simulink model "Problem_Iz"  (R2020b)
settings: Solver=VariableStepAuto  StartTime=0.0  StopTime=Ts  RelTol=1e-3
PreLoadFcn:
  | setUpPurePursuitCurveHighVel
model workspace (MAT data in the model file):
  firstWarning = 0
  originalScenarioChecksum = 'F73A6DA3C723D3CA73A6F931B7A52A9C'
values from neighbouring files (symbols this model uses):
  Cf = 34282    [matlab.mat]    (also in matlab2.mat)
  Cr = 34282    [matlab.mat]    (also in matlab2.mat)
  g = 9.81    [matlab.mat]    (also in matlab2.mat)
  i = 5.45    [matlab.mat]    (also in matlab2.mat)
  Iz = 162    [matlab.mat]    (also in matlab2.mat)
  L = 1.524    [matlab.mat]    (also in matlab2.mat)
  ld = 2    [matlab.mat]    (also in matlab2.mat)
  lf = 0.686    [matlab.mat]    (also in matlab2.mat)
  lr = 0.838    [matlab.mat]    (also in matlab2.mat)
  m = 300    [matlab.mat]    (also in matlab2.mat)
  Rw = 0.265    [matlab.mat]    (also in matlab2.mat)
  s = [73 1]    [matlab.mat]    (also in matlab2.mat)
  tr = 0.549    [matlab.mat]    (also in matlab2.mat)
  X_o = 0    [matlab.mat]    (also in matlab2.mat)
  xRef = [0 1.324067355 2.607903593 3.8125 4.901255524 5.841088879 6.603443704 7.165156233 7.509159117 7.625 7.509159117 7.165156233 ... (73 elements, 73x1)]    [matlab.mat]    (also in matlab2.mat)
  Y_o = 0    [matlab.mat]    (also in matlab2.mat)
  yRef = [0 0.115840883 0.459843767 1.021556296 1.783911121 2.723744476 3.8125 5.017096407 6.300932645 7.625 8.949067355 10.23290359 ... (73 elements, 73x1)]    [matlab.mat]    (also in matlab2.mat)
undefined symbols (not defined in the file or in its folder): psi_o, sigma1
libraries: autolibutils x4, autolibshared x3, simulink x3, pid_lib x2, vehdynlibviscommon x1, robotalgslib x1
(part 3 of 3)

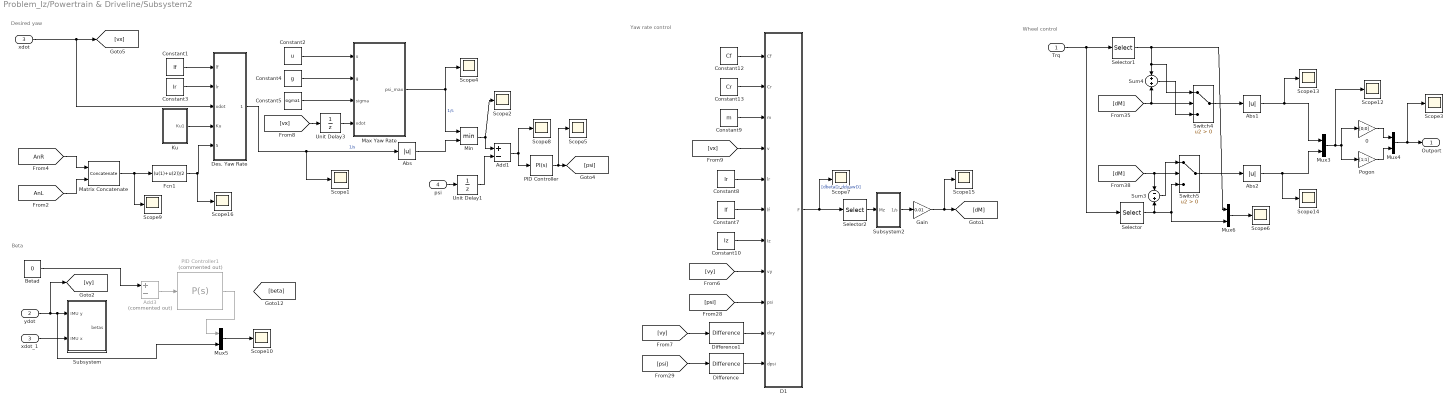
== system Problem_Iz/Powertrain & Driveline/Subsystem2 ==
  note: Desired yaw
  note: Beta
  note: Yaw rate control
  note: Wheel control
  Trq : Inport
  ydot : Inport  Port=2
  xdot : Inport  Port=3
  psi : Inport  Port=4
  0 : Gain  Gain=[0;0]
  Abs : Abs
  Abs1 : Abs
  Abs2 : Abs
  Add1 : Sum  Inputs=+-
  Add3 : Sum  Commented=on  Inputs=+-
  Betad : Constant  Value=0
  Constant1 : Constant  Value=lf
  Constant10 : Constant  Value=Iz
  Constant12 : Constant  Value=Cf
  Constant13 : Constant  Value=Cr
  Constant2 : Constant  Value=u
  Constant3 : Constant  Value=lr
  Constant4 : Constant  Value=g
  Constant5 : Constant  Value=sigma1
  Constant7 : Constant  Value=lf
  Constant8 : Constant  Value=lr
  Constant9 : Constant  Value=m
  D1 : MATLAB Function  TreatAsAtomicUnit=on
  Des. Yaw Rate : MATLAB Function  TreatAsAtomicUnit=on
  Difference : simulink/Discrete/Difference  ICPrevInput=0.0  OutMin=[]  OutMax=[]  OutDataType=fixdt(1, 16)  OutScaling=2^-10  DoSatur=off
  Difference1 : simulink/Discrete/Difference  ICPrevInput=0.0  OutMin=[]  OutMax=[]  OutDataType=fixdt(1, 16)  OutScaling=2^-10  DoSatur=off
  Fcn1 : Fcn  Expr=(u(1)+u(2))/2
  Gain : Gain  Gain=0.01
  Ku : Subsystem
  Matrix Concatenate : Concatenate
  Max Yaw Rate : MATLAB Function  TreatAsAtomicUnit=on
  Min : MinMax  Inputs=2
  Mux{3..6} (4 alike) : Mux  Inputs=2
  PID Controller : pid_lib/PID Controller  Controller=PI  Form=Parallel  TimeDomain=Continuous-time  UseExternalTs=off  SampleTime=-1  IntegratorMethod=Forward Euler  FilterMethod=Forward Euler  ControllerParametersSource=internal  P=4  I=12.5  D=0  UseFilter=on  N=100  TunerSelectOption=Transfer Function Based (PID Tuner App)  InitialConditionSource=internal  InitialConditionForIntegrator=0  InitialConditionForFilter=0  DifferentiatorICPrevScaledInput=0  ExternalReset=none  TrackingMode=off  Kt=1  LimitOutput=off  SatLimitsSource=internal  UpperSaturationLimit=inf  LowerSaturationLimit=-inf  LinearizeAsGain=on  AntiWindupMode=none  Kb=1  POutMin=[]  POutMax=[]  IOutMin=[]  IOutMax=[]  DOutMin=[]  DOutMax=[]  NOutMin=[]  NOutMax=[]  SumOutMin=[]  SumOutMax=[]  SaturationOutMin=[]  SaturationOutMax=[]  PParamMin=[]  PParamMax=[]  IParamMin=[]  IParamMax=[]  DParamMin=[]  DParamMax=[]  NParamMin=[]  NParamMax=[]  KbParamMin=[]  KbParamMax=[]  KtParamMin=[]  KtParamMax=[]  KbOutMin=[]  KbOutMax=[]  KtOutMin=[]  KtOutMax=[]  IntegratorOutMin=[]  IntegratorOutMax=[]  FilterOutMin=[]  FilterOutMax=[]  SumI1OutMin=[]  SumI1OutMax=[]  SumI2OutMin=[]  SumI2OutMax=[]  SumI3OutMin=[]  SumI3OutMax=[]  SumI4OutMin=[]  SumI4OutMax=[]  SumDOutMin=[]  SumDOutMax=[]  DifferentiatorOutMin=[]  DifferentiatorOutMax=[]  FilterDiffOutCoefMin=[]  FilterDiffOutCoefMax=[]  ReciprocalOutMin=[]  ReciprocalOutMax=[]  SumDenOutMin=[]  SumDenOutMax=[]  SumNumOutMin=[]  SumNumOutMax=[]  DivideOutMin=[]  DivideOutMax=[]  UdiffTsProdOutMin=[]  UdiffTsProdOutMax=[]  NTsProdOutMin=[]  NTsProdOutMax=[]  UintegralTsProdOutMin=[]  UintegralTsProdOutMax=[]  UngainTsProdOutMin=[]  UngainTsProdOutMax=[]  IntegratorContinuousStateAttributes=''  IntegratorStateMustResolveToSignalObject=off  IntegratorRTWStateStorageClass=Auto  FilterContinuousStateAttributes=''  FilterStateMustResolveToSignalObject=off  FilterRTWStateStorageClass=Auto  ParallelPVariant=InternalParameters  IdealPVariant=Disabled  IVariant=InternalParameters  DVariant=Disabled  IntegratorVariant=Continuous  SatVariant=Disabled  AWVariant=Passthrough  PCopyVariant=Disabled  TRVariant=Disabled  FdbkBlocksVariant=Forward  IdealPFdbkVariant=Disabled  SatFdbkVariant=Disabled  DerivativeFilterVariant=Disabled  NVariant=Disabled  NCopyVariant=Disabled_SignalSpec  FilterICVariant=Disabled  IntegratorICVariant=InternalICs  ExternalResetVariant=Disabled  TRSumVariant=Passthrough  SumFdbkVariant=Disabled  SumVariant=Sum_PI  TsampFilterVariant=InternalTs  TsampNgainVariant=Passthrough  TsampIntegralVariant=Passthrough  ExternalSaturationOutDataTypeStr=Inherit: Same as second input
  PID Controller1 : pid_lib/PID Controller  Commented=on  Controller=P  Form=Parallel  TimeDomain=Continuous-time  UseExternalTs=off  SampleTime=-1  IntegratorMethod=Forward Euler  FilterMethod=Forward Euler  ControllerParametersSource=internal  P=1  I=0.001  D=0  UseFilter=on  N=100  TunerSelectOption=Transfer Function Based (PID Tuner App)  InitialConditionSource=internal  InitialConditionForIntegrator=0  InitialConditionForFilter=0  DifferentiatorICPrevScaledInput=0  ExternalReset=none  TrackingMode=off  Kt=1  LimitOutput=off  SatLimitsSource=internal  UpperSaturationLimit=inf  LowerSaturationLimit=-inf  LinearizeAsGain=on  AntiWindupMode=none  Kb=1  POutMin=[]  POutMax=[]  IOutMin=[]  IOutMax=[]  DOutMin=[]  DOutMax=[]  NOutMin=[]  NOutMax=[]  SumOutMin=[]  SumOutMax=[]  SaturationOutMin=[]  SaturationOutMax=[]  PParamMin=[]  PParamMax=[]  IParamMin=[]  IParamMax=[]  DParamMin=[]  DParamMax=[]  NParamMin=[]  NParamMax=[]  KbParamMin=[]  KbParamMax=[]  KtParamMin=[]  KtParamMax=[]  KbOutMin=[]  KbOutMax=[]  KtOutMin=[]  KtOutMax=[]  IntegratorOutMin=[]  IntegratorOutMax=[]  FilterOutMin=[]  FilterOutMax=[]  SumI1OutMin=[]  SumI1OutMax=[]  SumI2OutMin=[]  SumI2OutMax=[]  SumI3OutMin=[]  SumI3OutMax=[]  SumI4OutMin=[]  SumI4OutMax=[]  SumDOutMin=[]  SumDOutMax=[]  DifferentiatorOutMin=[]  DifferentiatorOutMax=[]  FilterDiffOutCoefMin=[]  FilterDiffOutCoefMax=[]  ReciprocalOutMin=[]  ReciprocalOutMax=[]  SumDenOutMin=[]  SumDenOutMax=[]  SumNumOutMin=[]  SumNumOutMax=[]  DivideOutMin=[]  DivideOutMax=[]  UdiffTsProdOutMin=[]  UdiffTsProdOutMax=[]  NTsProdOutMin=[]  NTsProdOutMax=[]  UintegralTsProdOutMin=[]  UintegralTsProdOutMax=[]  UngainTsProdOutMin=[]  UngainTsProdOutMax=[]  IntegratorContinuousStateAttributes=''  IntegratorStateMustResolveToSignalObject=off  IntegratorRTWStateStorageClass=Auto  FilterContinuousStateAttributes=''  FilterStateMustResolveToSignalObject=off  FilterRTWStateStorageClass=Auto  ParallelPVariant=InternalParameters  IdealPVariant=Disabled  IVariant=Disabled  DVariant=Disabled  IntegratorVariant=Disabled  SatVariant=Disabled  AWVariant=Disabled  PCopyVariant=Disabled  TRVariant=Disabled  FdbkBlocksVariant=Forward  IdealPFdbkVariant=Disabled  SatFdbkVariant=Disabled  DerivativeFilterVariant=Disabled  NVariant=Disabled  NCopyVariant=Disabled_SignalSpec  FilterICVariant=Disabled  IntegratorICVariant=Disabled  ExternalResetVariant=Disabled  TRSumVariant=Passthrough  SumFdbkVariant=Disabled  SumVariant=Passthrough_P  TsampFilterVariant=InternalTs  TsampNgainVariant=Passthrough  TsampIntegralVariant=Disabled_SignalSpec  ExternalSaturationOutDataTypeStr=Inherit: Same as second input
  Pogon : Gain  Gain=[1;1]
  Scope{1..10,12..16} (15 alike) : Scope
  Selector : Selector  InputPortWidth=4  IndexOptions=Index vector (dialog)  Indices=[4 ]  OutputSizes=1
  Selector1 : Selector  InputPortWidth=4  IndexOptions=Index vector (dialog)  Indices=[3]  OutputSizes=1
  Selector2 : Selector  InputPortWidth=2  IndexOptions=Index vector (dialog)  Indices=[1]  OutputSizes=1
  Subsystem : Subsystem
  Subsystem2 : Subsystem
  Sum3 : Sum  Inputs=-+
  Sum4 : Sum
  Switch4 : Switch  Criteria=u2 > Threshold
  Switch5 : Switch  Criteria=u2 > Threshold
  Unit Delay1 : UnitDelay  SampleTime=0.7  HasFrameUpgradeWarning=on
  Unit Delay3 : UnitDelay  SampleTime=0.7  HasFrameUpgradeWarning=on
  xdot_1 : InportShadow  Port=3
  Outport : Outport
  wires:
  [psi] -> D1/9(psi)
  [AnR] -> Matrix Concatenate/1
  Constant12/1 -> D1/1(Cf)
  Trq/1 -> Selector/1, Selector1/1
  xdot/1 -> [vx], Des. Yaw Rate/3(xdot)
  [AnL] -> Matrix Concatenate/2
  Constant3/1 -> Des. Yaw Rate/2(lr)
  psi/1 -> Unit Delay1/1
  Constant4/1 -> Max Yaw Rate/2(g)
  [vy] -> Difference1/1
  Des. Yaw Rate/1(psi_des) -> Abs/1, Scope1/1  "1/s"
  [vx] -> D1/4(v)
  Constant2/1 -> Max Yaw Rate/1(u)
  Mux3/1 -> Scope12/1, 0/1, Pogon/1
  Matrix Concatenate/1 -> Scope9/1, Fcn1/1
  D1/1(F) -> Selector2/1, Scope7/1  "[dbetaD; ddyawD]"
  Constant5/1 -> Max Yaw Rate/3(sigma)
  [psi] -> Difference/1
  Switch5/1 -> Abs2/1
  Min/1 -> Add1/1, Scope2/1
  [dM] -> Switch5/2, Sum3/1
  Sum3/1 -> Switch5/1
  Mux4/1 -> Outport/1, Scope3/1
  Constant13/1 -> D1/2(Cr)
  Constant8/1 -> D1/5(lr)
  Constant9/1 -> D1/3(m)
  Constant7/1 -> D1/6(lf)
  0/1 -> Mux4/1
  Constant1/1 -> Des. Yaw Rate/1(lf)
  Fcn1/1 -> Scope16/1, Des. Yaw Rate/5(WhiAngF)
  Betad/1 -> Add3/1
  PID Controller/1 -> Scope5/1, [psi]
  [dM] -> Sum4/2, Switch4/2
  Max Yaw Rate/1(psi_max) -> Min/1, Scope4/1  "1/s"
  [vy] -> D1/8(vy)
  Selector/1 -> Mux6/2, Switch5/3, Sum3/2
  PID Controller1/1 -> Mux5/1
  Sum4/1 -> Switch4/3
  Ku/1(Ku1) -> Des. Yaw Rate/4(Ku)
  ydot/1 -> [vy], Mux5/2, Subsystem/1(IMU y)
  Constant10/1 -> D1/7(Iz)
  Add3/1 -> PID Controller1/1
  [vx] -> Unit Delay3/1
  xdot_1/1 -> Subsystem/2(IMU x)
  Pogon/1 -> Mux4/2
  Selector1/1 -> Mux6/1, Switch4/1, Sum4/1
  Switch4/1 -> Abs1/1
  Mux5/1 -> Scope10/1
  Mux6/1 -> Scope6/1
  Unit Delay3/1 -> Max Yaw Rate/4(xdot)
  Add1/1 -> Scope8/1, PID Controller/1
  Abs/1 -> Min/2
  Difference1/1 -> D1/10(dvy)
  Difference/1 -> D1/11(dpsi)
  Selector2/1 -> Subsystem2/1(Mz)
  Unit Delay1/1 -> Add1/2
  Subsystem2/1(1/s) -> Gain/1
  Abs1/1 -> Mux3/1, Scope13/1
  Abs2/1 -> Scope14/1, Mux3/2
  Gain/1 -> Scope15/1, [dM]

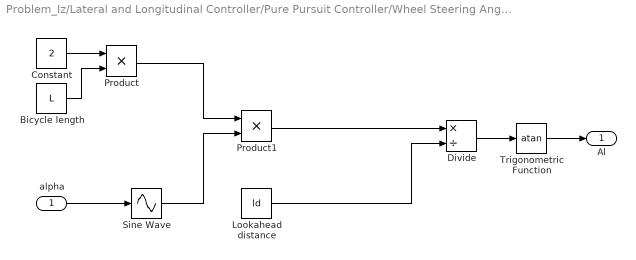
== system Problem_Iz/Lateral and Longitudinal Controller/Pure Pursuit Controller/Wheel Steering Angle Formulation ==
  alpha : Inport
  Bicycle length : Constant  Value=L
  Constant : Constant  Value=2
  Divide : Product  Inputs=*/
  Lookahead distance : Constant  Value=ld
  Product : Product
  Product1 : Product
  Sine Wave : Sin  TimeSource=Use external signal  SampleTime=0
  Trigonometric Function : Trigonometry  Operator=atan
  Al : Outport
  wires:
  Sine Wave/1 -> Product1/2
  Bicycle length/1 -> Product/2
  Constant/1 -> Product/1
  Product1/1 -> Divide/1
  Product/1 -> Product1/1
  Divide/1 -> Trigonometric Function/1
  Trigonometric Function/1 -> Al/1
  alpha/1 -> Sine Wave/1
  Lookahead distance/1 -> Divide/2

== system Problem_Iz/Powertrain & Driveline/Driveline/RWD ==
  TPowertrain : Inport
  RWD : Gain  Gain=[0;0;1;1]
  TAxles : Outport  VectorParamsAs1DForOutWhenUnconnected=off
  wires:
  TPowertrain/1 -> RWD/1
  RWD/1 -> TAxles/1

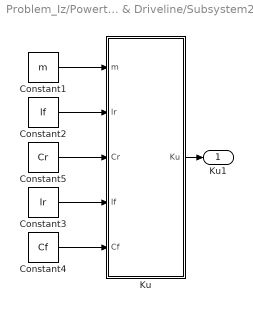
== system Problem_Iz/Powertrain & Driveline/Subsystem2/Ku ==
  Constant1 : Constant  Value=m
  Constant2 : Constant  Value=lf
  Constant3 : Constant  Value=lr
  Constant4 : Constant  Value=Cf
  Constant5 : Constant  Value=Cr
  Ku : MATLAB Function  TreatAsAtomicUnit=on
  Ku1 : Outport
  wires:
  Ku/1(Ku) -> Ku1/1
  Constant5/1 -> Ku/3(Cr)
  Constant2/1 -> Ku/2(lr)
  Constant3/1 -> Ku/4(lf)
  Constant1/1 -> Ku/1(m)
  Constant4/1 -> Ku/5(Cf)

== system Problem_Iz/Powertrain & Driveline/Subsystem2/Subsystem ==
  IMU y : Inport
  IMU x : Inport  Port=2
  Betas : Product  Inputs=*/
  Scope1 : Scope
  Tan : Trigonometry  Operator=atan
  betas : Outport
  wires:
  IMU y/1 -> Betas/1
  IMU x/1 -> Betas/2
  Betas/1 -> Tan/1
  Tan/1 -> Scope1/1, betas/1

== system Problem_Iz/Powertrain & Driveline/Subsystem2/Subsystem2 ==
  Mz : Inport
  Constant11 : Constant  Value=i
  Constant14 : Constant  Value=tr
  Constant6 : Constant  Value=Rw
  Des. Yaw Rate1 : MATLAB Function  TreatAsAtomicUnit=on
  1/s : Outport
  wires:
  Des. Yaw Rate1/1(dM) -> 1/s/1  "1/s"
  Constant14/1 -> Des. Yaw Rate1/3(tr)
  Constant6/1 -> Des. Yaw Rate1/1(Rw)
  Mz/1 -> Des. Yaw Rate1/4(Mz)
  Constant11/1 -> Des. Yaw Rate1/2(i)

== matlab function Problem_Iz/Powertrain & Driveline/Subsystem2/Ku/Ku ==
  data: m input; Ku output; lr input; Cr input; lf input; Cf input
function Ku = fcn(m, lr, Cr, lf, Cf)
%#codegen

Ku = (lr*m)/((lf+lr)^2 *Cf)-(lf*m)/((lf+lr)^2 *Cr);

== matlab function Problem_Iz/Powertrain & Driveline/Subsystem2/D1 ==
  data: Cf input; F output; Cr input; m input; v input; lr input; lf input; Iz input; vy input; psi input; dvy input; dpsi input
function F = fcn(Cf, Cr, m, v, lr, lf, Iz, vy, psi,dvy, dpsi)

A11 = (-Cf - Cr)/(m*v);
A12 = - 1 + (Cr*lr - Cf*lf)/(m*v^2);
A21 = (Cr*lr - Cf*lf)/(Iz*v);
A22 = (-Cf*lf^2 - Cr*lr^2)/(Iz*v);
A = [[A11, A12]; [A21, A22]];

B1 = vy;
B2 = psi;
x = [B1; B2];

D1 = dvy;
D2 = dpsi;
D = [D1; D2];

C11 = -lf * m;
C12 = Iz;
C21 = m/Cf;
C22 = 0;
C = [C11 C12; C21 C22];

F = C*(D - A*x);

== matlab function Problem_Iz/Powertrain & Driveline/Subsystem2/Max Yaw Rate ==
  data: u input; psi_max output; g input; sigma input; xdot input
function psi_max = fcn(u, g, sigma, xdot)
%#codegen


psi_max = sigma * g * u / xdot;

== matlab function Problem_Iz/Powertrain & Driveline/Side Slip Angle1 ==
  data: lf input; R output; lr input; Cf input; Cr input; m input; vx input; Iz input; sigma input; vy input; psi input; Mz input
function R = fcn(lf, lr, Cf, Cr, m, vx, Iz, sigma, vy, psi, Mz)
%#codegen

A11 = (- Cf - Cr)/( m*vx );
A12 = - vx + (-Cf*lf + Cr*lr)/(m*vx);
A21 = (-Cf*lf + Cr*lr)/(Iz*vx);
A22 = (-Cf*lf^2 - Cr*lr^2)/(Iz*vx);
A = [A11 A12; A21 A22];

E11 = 0;
E12 = Cf/m;
E21 = 1/Iz;
E22 = lf*Cf/Iz;
E = [E11 E12; E21 E22];

x = [vy; psi];

y = [Mz; sigma];

R = A*x + E*y;

== matlab function Problem_Iz/Powertrain & Driveline/Subsystem2/Des. Yaw Rate ==
  data: lf input; psi_des output; lr input; xdot input; Ku input; WhiAngF input
function psi_des = fcn( lf, lr , xdot, Ku, WhiAngF)
%#codegen


psi_des = xdot/((lf + lr) + Ku * xdot^2) * WhiAngF;

== matlab function Problem_Iz/Powertrain & Driveline/Subsystem2/Subsystem2/Des. Yaw Rate1 ==
  data: Rw input; dM output; i input; tr input; Mz input
function dM = fcn( Rw, i, tr, Mz)
%#codegen


dM = Mz * Rw / (2 * i * tr);
